simulink model "modelagem"  (R2018b)
settings: Solver=VariableStepAuto  StartTime=0.0  StopTime=3  RelTol=1e-3
settings Model: Creator=bernardo  LastModifiedBy=bernardo

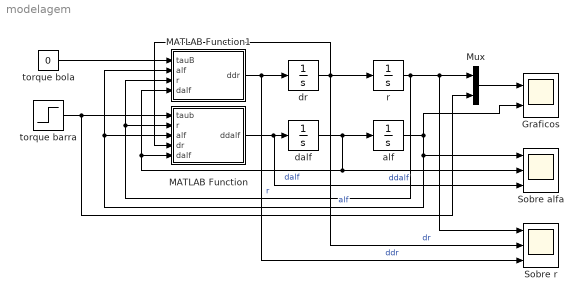
== system modelagem ==
  Graficos : Scope  NumInputPorts=2
  MATLAB Function : MATLAB Function  TreatAsAtomicUnit=on
  MATLAB Function1 : MATLAB Function  TreatAsAtomicUnit=on
  Mux : Mux  Inputs=2
  Sobre alfa : Scope  NumInputPorts=3
  Sobre r : Scope  NumInputPorts=3
  alf : Integrator
  dalf : Integrator
  dr : Integrator
  r : Integrator
  torque barra : Step  Time=0  SampleTime=0.001
  torque bola : Constant  Value=0
  wires:
  torque barra/1 -> Mux/2, MATLAB Function/1(taub)
  torque bola/1 -> MATLAB Function1/1(tauB)
  MATLAB Function/1(ddalf) -> Sobre alfa/3, dalf/1  "ddalf"
  dalf/1 -> MATLAB Function/5(dalf), MATLAB Function1/4(dalf), Sobre alfa/2, alf/1  "dalf"
  alf/1 -> Graficos/2, MATLAB Function/3(alf), MATLAB Function1/2(alf), Sobre alfa/1  "alf"
  MATLAB Function1/1(ddr) -> dr/1, Sobre r/3  "ddr"
  dr/1 -> r/1, MATLAB Function/4(dr), Sobre r/2  "dr"
  r/1 -> MATLAB Function1/3(r), MATLAB Function/2(r), Sobre r/1, Mux/1  "r"
  Mux/1 -> Graficos/1

== matlab function modelagem/MATLAB Function1 ==
  data: tauB input; ddr output; alf input; r input; dalf input
function ddr = fnc(tauB, alf, r, dalf)
    mB = 3e-3;
    g  = 9.8;
    R = 20e-3;
    JB = 2/5*mB*R^2;
    
    
%     mB = 0.0282;    % kg
%     R  = 0.0095;    % m
%     JB = 1.0469e-6; % kg*m^2
%     g  = 9.8;       % m/s^2


    a = mB + JB/R^2;
ddr = 1/a * ( tauB + mB*r*dalf^2 - mB*g*sin(alf) );

== matlab function modelagem/MATLAB Function ==
  data: taub input; ddalf output; r input; alf input; dr input; dalf input
function ddalf = fcn(taub, r, alf, dr, dalf)
    mB = 3e-3;
    mb = 2;
    R = 20e-3;
    L  = 400e-3;
    JB = 2/5*mB*R^2;
    Jb = 1/12*mb*( 3*(8e-3)^2 + 4*L^2);
    g  = 9.8;

%     mB = 0.0282;    % kg
%     mb = 0.334;     % kg
%     L  = 0.4;       % m
%     JB = 1.0469e-6; % kg*m^2
%     Jb = 0.017813;  % kg*m^2
%     g  = 9.8;       % m/s^2

    

    b = mB*r^2 + JB + Jb;
    y = 1/b * (taub - 2*mB*r*dr*dalf - g*(0.5*L*mb + mB*r)*cos(alf) );
ddalf = y;
